simulink model "model6_ExtendedEstimator"  (R2020a)
settings: Solver=FixedStepAuto  StartTime=0.0  StopTime=T  FixedStep=Ts  RelTol=1e-3
undefined symbols (not defined in the file): alpha0, alpha1, K, Lz, omgn, rFlag, Ts, wFlag, x0
settings Model: Creator=XiaoCY  LastModifiedBy=XiaoCY
settings DataIOCC: ReturnWorkspaceOutputs=off

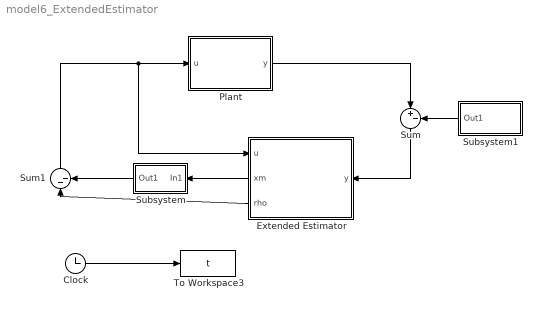
== system model6_ExtendedEstimator ==
  Clock : Clock
  Extended Estimator : Subsystem
      settings: PortSchema="{\"entries\":[{\"content\":{\"sides\":[{\"content\":{\"connectorIds\":[\"In1\"]},\"type\":\"ConnectorPlacement.EquallySpacedRectSide\",\"uuid\":\"995efd48-3db5-4a6e-85f6-a349d6a63930\"},{\"content\":{\"connectorIds\":[\"In2\",\"Out1\",\"Out2\"],\"side\":\"RIGHT\"},\"type\":\"ConnectorPlacement.EquallySpacedRectSide\",\"uuid\":\"626e22d4-5752-4239-b2ce-472c77ace920\"},{\"content\":{\"connectorIds\":[],\"side\":\"TOP\"},\"type\":\"ConnectorPlacement.EquallySpacedRectSide\",\"uuid\":\"cb599412-420c-4014-940e-49f432b7cbea\"}]},\"type\":\"ConnectorPlacement.EquallySpacedConnector\",\"uuid\":\"e0cccee1-86a0-41f4-a3e5-9044b1b28e69\"}],\"packageUris\":[\"http://schema.mathworks.com/mf0/Connector/19700101\"],\"version\":\"1.0\"}"
  Plant : Subsystem
  Subsystem : Subsystem
      mask Display: disp('Kx')
  Subsystem1 : Subsystem
      mask Display: disp('Reference')
  Sum : Sum  Inputs=|+-
  Sum1 : Sum  Inputs=|--
  To Workspace3 : ToWorkspace  VariableName=t  SampleTime=Ts
  wires:
  Plant/1(y) -> Sum/1
  Extended Estimator/1(xm) -> Subsystem/1(In1)
  Sum/1 -> Extended Estimator/1(y)
  Subsystem1/1(Out1) -> Sum/2
  Subsystem/1(Out1) -> Sum1/2
  Extended Estimator/2(rho) -> Sum1/1
  Sum1/1 -> Extended Estimator/2(u), Plant/1(u)
  Clock/1 -> To Workspace3/1

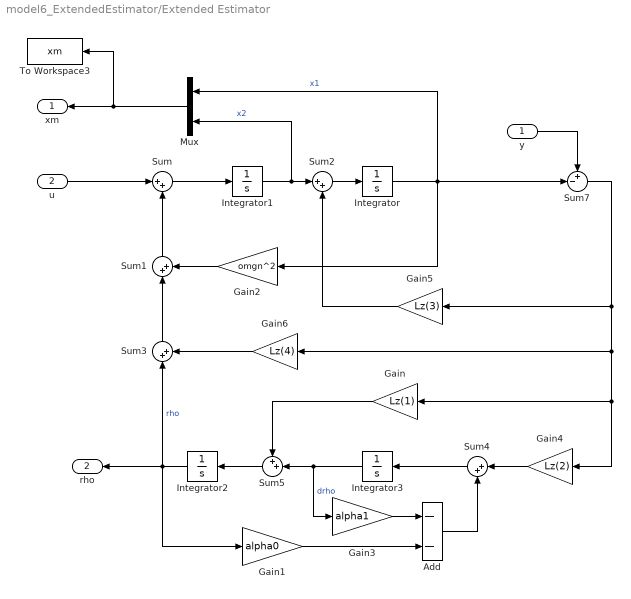
== system model6_ExtendedEstimator/Extended Estimator ==
  y : Inport
  u : Inport  Port=2
  Add : Sum  Inputs=--
  Gain : Gain  Gain=Lz(1)
  Gain1 : Gain  Gain=alpha0
  Gain2 : Gain  Gain=omgn^2
  Gain3 : Gain  Gain=alpha1
  Gain4 : Gain  Gain=Lz(2)
  Gain5 : Gain  Gain=Lz(3)
  Gain6 : Gain  Gain=Lz(4)
  Integrator{,1..3} (4 alike) : Integrator
  Mux : Mux  Inputs=2
  Sum{,1..4} (5 alike) : Sum  Inputs=|++
  Sum5 : Sum  Inputs=++|
  Sum7 : Sum  Inputs=+-|
  To Workspace3 : ToWorkspace  VariableName=xm  SampleTime=Ts
  xm : Outport
  rho : Outport  Port=2
  wires:
  Integrator/1 -> Gain2/1, Mux/1, Sum7/2  "x1"
  Integrator1/1 -> Mux/2, Sum2/1  "x2"
  Integrator3/1 -> Sum5/2, Gain3/1  "drho"
  Integrator2/1 -> Sum3/1, rho/1, Gain1/1  "rho"
  u/1 -> Sum/1
  Gain3/1 -> Add/1
  Gain1/1 -> Add/2
  Add/1 -> Sum4/2
  Sum/1 -> Integrator1/1
  Sum2/1 -> Integrator/1
  Sum5/1 -> Integrator2/1
  y/1 -> Sum7/1
  Sum4/1 -> Integrator3/1
  Mux/1 -> To Workspace3/1, xm/1
  Sum1/1 -> Sum/2
  Gain/1 -> Sum5/1
  Gain4/1 -> Sum4/1
  Gain2/1 -> Sum1/2
  Sum3/1 -> Sum1/1
  Gain6/1 -> Sum3/2
  Gain5/1 -> Sum2/2
  Sum7/1 -> Gain4/1, Gain/1, Gain6/1, Gain5/1

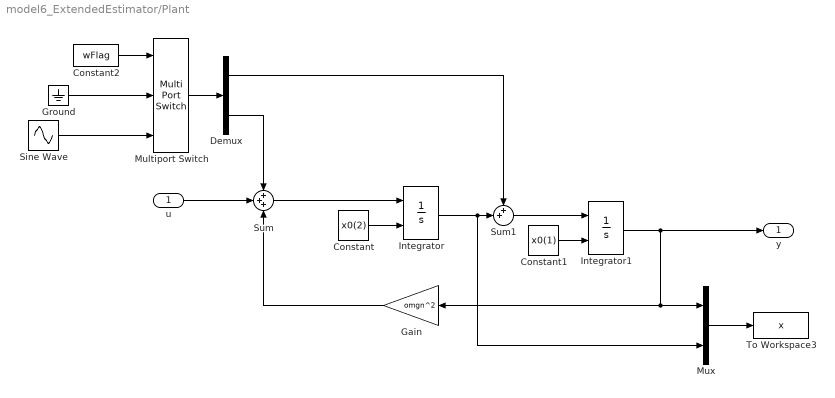
== system model6_ExtendedEstimator/Plant ==
  u : Inport
  Constant : Constant  Value=x0(2)
  Constant1 : Constant  Value=x0(1)
  Constant2 : Constant  Value=wFlag
  Demux : Demux  Outputs=2
  Gain : Gain  Gain=omgn^2
  Ground : Ground
  Integrator : Integrator  InitialConditionSource=external
  Integrator1 : Integrator  InitialConditionSource=external
  Multiport Switch : MultiPortSwitch  DataPortOrder=Zero-based contiguous  Inputs=2  zeroidx=on
  Mux : Mux  Inputs=2
  Sine Wave : Sin  Amplitude=[3 5]  Frequency=alpha0  Phase=[30 60]  SampleTime=0
  Sum : Sum  Inputs=+++
  Sum1 : Sum  Inputs=++|
  To Workspace3 : ToWorkspace  VariableName=x  SampleTime=Ts
  y : Outport
  wires:
  Integrator/1 -> Sum1/2, Mux/2
  Constant1/1 -> Integrator1/2
  u/1 -> Sum/2
  Constant/1 -> Integrator/2
  Sum/1 -> Integrator/1
  Gain/1 -> Sum/3
  Mux/1 -> To Workspace3/1
  Integrator1/1 -> Gain/1, Mux/1, y/1
  Constant2/1 -> Multiport Switch/1
  Ground/1 -> Multiport Switch/2
  Sine Wave/1 -> Multiport Switch/3
  Multiport Switch/1 -> Demux/1
  Demux/2 -> Sum/1
  Sum1/1 -> Integrator1/1
  Demux/1 -> Sum1/1

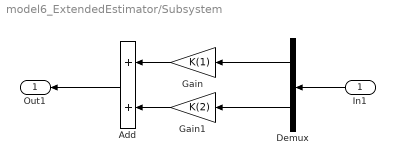
== system model6_ExtendedEstimator/Subsystem ==
  In1 : Inport
  Add : Sum
  Demux : Demux  Outputs=2
  Gain : Gain  Gain=K(1)
  Gain1 : Gain  Gain=K(2)
  Out1 : Outport
  wires:
  In1/1 -> Demux/1
  Add/1 -> Out1/1
  Gain/1 -> Add/1
  Gain1/1 -> Add/2
  Demux/1 -> Gain/1
  Demux/2 -> Gain1/1

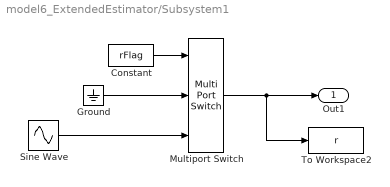
== system model6_ExtendedEstimator/Subsystem1 ==
  Constant : Constant  Value=rFlag
  Ground : Ground
  Multiport Switch : MultiPortSwitch  DataPortOrder=Zero-based contiguous  Inputs=2  zeroidx=on
  Sine Wave : Sin  Frequency=alpha0  SampleTime=0
  To Workspace2 : ToWorkspace  VariableName=r  SampleTime=Ts
  Out1 : Outport
  wires:
  Sine Wave/1 -> Multiport Switch/3
  Multiport Switch/1 -> To Workspace2/1, Out1/1
  Ground/1 -> Multiport Switch/2
  Constant/1 -> Multiport Switch/1
